simulink model "Three_order_noliner1"  (R2023a)
settings: Solver=VariableStepAuto  StartTime=0.0  StopTime=1000  FixedStep=1  RelTol=1e-3
values from neighbouring files (symbols this model uses):
  c0 = 1.128    [analysis_com.m]
  c1 = bestParams(1)    [analysis_com.m]
  c2 = bestParams(2)    [analysis_com.m]
  d1 = bestParams(3)    [analysis_com.m]
  d2 = bestParams(4)    [analysis_com.m]
  hfw = 1200    [analysis_com.m]
settings Model: Creator=Administrator  LastModifiedBy=鲁宇轩
settings DebuggingCC: UnconnectedInputMsg=warning  UnconnectedOutputMsg=warning  UnconnectedLineMsg=warning
settings ModelReferenceCC: EnableRefExpFcnMdlSchedulingChecks=on
settings RTWCC: DLArmComputeVersion=19.05

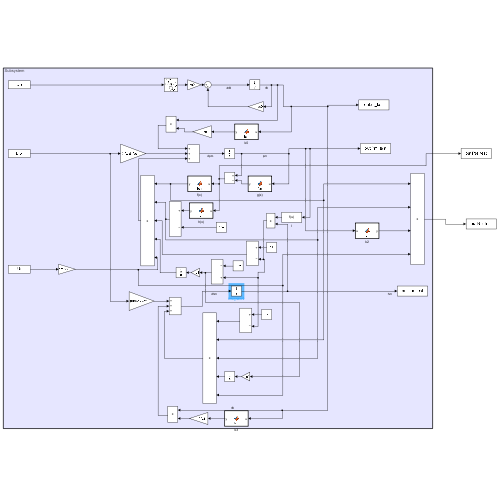
[thumbnail: Simulink's stored preview of the top-level diagram]
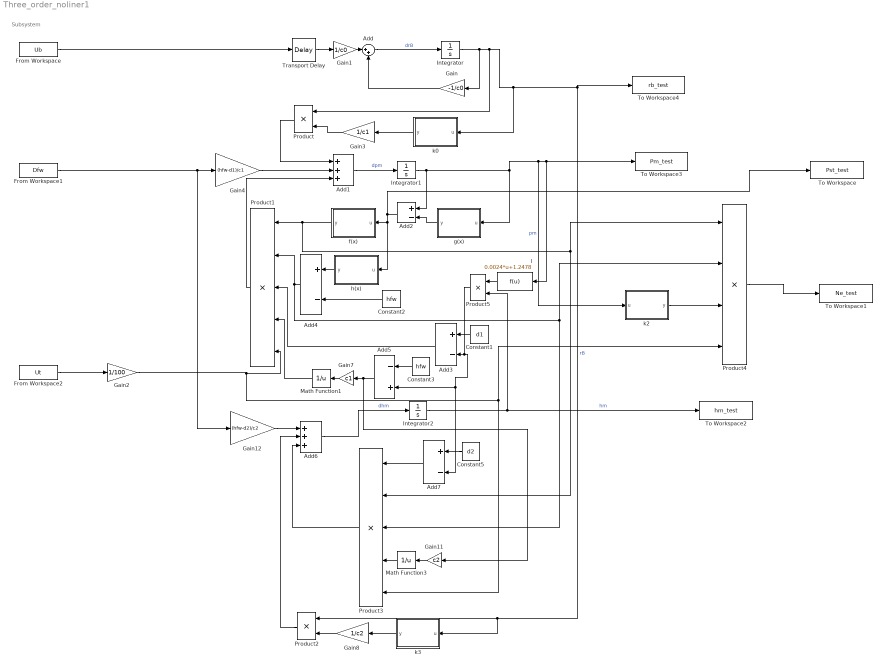
== system Three_order_noliner1 ==
  note: Subsystem
  Add : Sum  Inputs=|++
  Add1 : Sum  Inputs=+++
  Add{2..4,7} (4 alike) : Sum  Inputs=+-
  Add5 : Sum  Inputs=-+
  Add6 : Sum  Inputs=+++
  Constant1 : Constant  Value=d1
  Constant2 : Constant  Value=hfw
  Constant3 : Constant  Value=hfw
  Constant5 : Constant  Value=d2
  From Workspace : FromWorkspace  VariableName=Ub
  From Workspace1 : FromWorkspace  VariableName=Dfw
  From Workspace2 : FromWorkspace  VariableName=Ut
  Gain : Gain  Gain=-1/c0
  Gain1 : Gain  Gain=1/c0
  Gain11 : Gain  Gain=c2
  Gain12 : Gain  Gain=(hfw-d2)/c2
  Gain2 : Gain  Gain=1/100
  Gain3 : Gain  Gain=1/c1
  Gain4 : Gain  Gain=(hfw-d1)/c1
  Gain7 : Gain  Gain=c1
  Gain8 : Gain  Gain=1/c2
  Integrator : Integrator  InitialCondition=181.63
  Integrator1 : Integrator  InitialCondition=24
  Integrator2 : Integrator  InitialCondition=2441.5
  Math Function1 : Math  Operator=reciprocal
  Math Function3 : Math  Operator=reciprocal
  Product : Product
  Product1 : Product  Inputs=5
  Product2 : Product
  Product3 : Product  Inputs=5
  Product4 : Product  Inputs=4
  Product5 : Product
  To Workspace : ToWorkspace  VariableName=Pst_test  SaveFormat=Timeseries  SampleTime=1
  To Workspace1 : ToWorkspace  VariableName=Ne_test  SaveFormat=Timeseries  SampleTime=1
  To Workspace2 : ToWorkspace  VariableName=hm_test  SaveFormat=Timeseries  SampleTime=1
  To Workspace3 : ToWorkspace  VariableName=Pm_test  SaveFormat=Timeseries  SampleTime=1
  To Workspace4 : ToWorkspace  VariableName=rb_test  SaveFormat=Timeseries  SampleTime=1
  Transport Delay : TransportDelay  DelayTime=t  InitialOutput=182.31
  f(x) : MATLAB Function  TreatAsAtomicUnit=on
  g(x) : MATLAB Function  TreatAsAtomicUnit=on
  h(x) : MATLAB Function  TreatAsAtomicUnit=on
  k0 : MATLAB Function  TreatAsAtomicUnit=on
  k2 : MATLAB Function  TreatAsAtomicUnit=on
  k3 : MATLAB Function  TreatAsAtomicUnit=on
  l : Fcn  Expr=0.0024*u+1.2478
  wires:
  Gain2/1 -> Product4/4, Product3/5, Product1/5
  Gain8/1 -> Product2/2
  Product3/1 -> Add6/3
  Product2/1 -> Add6/2
  Math Function1/1 -> Product1/4
  g(x)/1(y) -> Add2/2
  From Workspace/1 -> Transport Delay/1
  Gain3/1 -> Product/2
  Gain12/1 -> Add6/1
  Add6/1 -> Integrator2/1  "dhm"
  Add3/1 -> Product1/3
  k2/1(y) -> Product4/3
  Add7/1 -> Product3/1
  Constant1/1 -> Add3/1
  h(x)/1(y) -> Add4/1
  From Workspace1/1 -> Gain4/1, Gain12/1
  Constant3/1 -> Add5/1
  Constant5/1 -> Add7/1
  f(x)/1(y) -> Product3/2, Product4/1, Product1/1
  Gain1/1 -> Add/1
  Add/1 -> Integrator/1  "drB"
  Product/1 -> Add1/1
  Gain7/1 -> Math Function1/1
  Integrator1/1 -> g(x)/1(u), l/1, To Workspace3/1, k2/1(u), Add2/1  "pm"
  Product4/1 -> To Workspace1/1
  Product1/1 -> Add1/3
  Transport Delay/1 -> Gain1/1
  Gain4/1 -> Add1/2
  Constant2/1 -> Add4/2
  Gain/1 -> Add/2
  Add1/1 -> Integrator1/1  "dpm"
  From Workspace2/1 -> Gain2/1
  Gain11/1 -> Math Function3/1
  Add5/1 -> Gain11/1, Gain7/1
  Add4/1 -> Product3/3, Product4/2, Product1/2
  Integrator2/1 -> To Workspace2/1, Product5/2  "hm"
  Integrator/1 -> Gain/1, Product/1, k0/1(u), k3/1(u), Product2/1, To Workspace4/1  "rB"
  Math Function3/1 -> Product3/4
  k0/1(y) -> Gain3/1
  k3/1(y) -> Gain8/1
  Add2/1 -> To Workspace/1, h(x)/1(u), f(x)/1(u)
  l/1 -> Product5/1
  Product5/1 -> Add3/2, Add7/2, Add5/2

== matlab function Three_order_noliner1/g(x) ==
  data: u input; y output
function y = fcn(u)
y = 0.0709*u-0.0116;
end

== matlab function Three_order_noliner1/h(x) ==
  data: u input; y output
function y = fcn(u)

y =-11.116*u+3616.5;

== matlab function Three_order_noliner1/k0 ==
  data: u input; y output
function y = fcn(u)
y = -13.8951*u+12747;
end

== matlab function Three_order_noliner1/k2 ==
  data: u input; y output
function y = fcn(u)
y = (1.25e-6)*u+(1.28e-4);
end

== matlab function Three_order_noliner1/k3 ==
  data: u input; y output
function y = fcn(u)
y =-13.9851*u+12747;
end

== matlab function Three_order_noliner1/f(x) ==
  data: u input; y output
function y = fcn(u)
y =48.213*u-17.68;
end
